simulink model "springmassdamper"  (R2019a)
settings: Solver=ode4  StartTime=0.0  StopTime=5  FixedStep=0.001  RelTol=1e-3
values from neighbouring files (symbols this model uses):
  c = 2 * m * nat_f * 0.05    [smyth_project_2.m]
  k = 19990    [smyth_project_2.m]
  m = 23    [smyth_project_2.m]
  nat_f = sqrt(k/m)    [smyth_project_2.m]
  run_case = 5    [smyth_project_2.m]
  x0 = 0    [smyth_project_2.m]
settings Model: Creator=crsmyth  LastModifiedBy=Ross

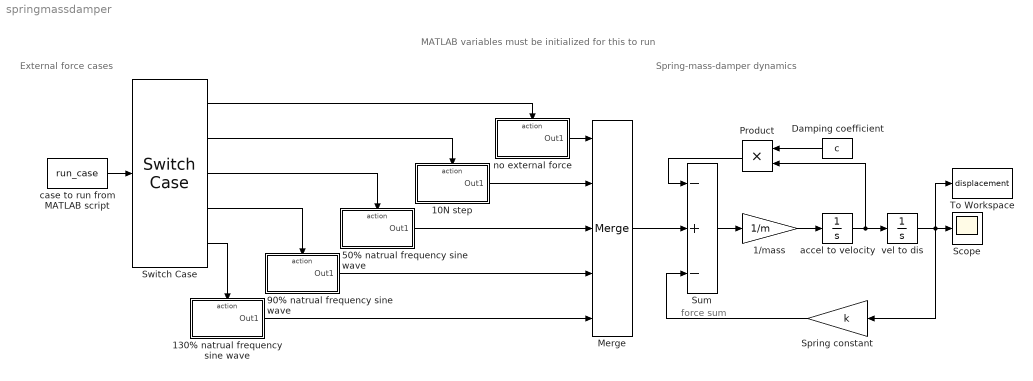
== system springmassdamper ==
  note: MATLAB variables must be initialized for this to run
  note: Spring-mass-damper dynamics
  note: External force cases
  note: force sum
  1/mass : Gain  Gain=1/m
  10N step : Subsystem  TreatAsAtomicUnit=on
  130% natrual frequency sine wave : Subsystem  TreatAsAtomicUnit=on
  50% natrual frequency sine wave : Subsystem  TreatAsAtomicUnit=on
  90% natrual frequency sine wave : Subsystem  TreatAsAtomicUnit=on
  Damping coefficient : Constant  Value=c
  Merge : Merge  Inputs=5
  Product : Product
  Scope : Scope
  Spring constant : Gain  Gain=k
  Sum : Sum  Inputs=-+-
  Switch Case : SwitchCase  CaseConditions={1, 2, 3, 4, 5}  ShowDefaultCase=off
  To Workspace : ToWorkspace  VariableName=displacement  SampleTime=-1
      settings: Save2DSignal=2-D array (concatenate along first dimension)
  accel to velocity : Integrator
  case to run from MATLAB script : Constant  Value=run_case
  no external force : Subsystem  TreatAsAtomicUnit=on
  vel to dis : Integrator  InitialCondition=x0
  wires:
  Sum/1 -> 1/mass/1
  vel to dis/1 -> Scope/1, Spring constant/1, To Workspace/1
  Merge/1 -> Sum/2
  accel to velocity/1 -> Product/2, vel to dis/1
  1/mass/1 -> accel to velocity/1
  Spring constant/1 -> Sum/3
  Switch Case/1 -> no external force/Action
  case to run from MATLAB script/1 -> Switch Case/1
  no external force/1(Out1) -> Merge/1
  10N step/1(Out1) -> Merge/2
  Switch Case/2 -> 10N step/Action
  50% natrual frequency sine wave/1(Out1) -> Merge/3
  Switch Case/3 -> 50% natrual frequency sine wave/Action
  90% natrual frequency sine wave/1(Out1) -> Merge/4
  Switch Case/4 -> 90% natrual frequency sine wave/Action
  130% natrual frequency sine wave/1(Out1) -> Merge/5
  Switch Case/5 -> 130% natrual frequency sine wave/Action
  Product/1 -> Sum/1
  Damping coefficient/1 -> Product/1

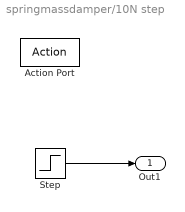
== system springmassdamper/10N step ==
  Action Port : ActionPort  ActionPortLabel=case [ 2 ]:
  Step : Step  Time=0  After=10  SampleTime=0
  Out1 : Outport
  wires:
  Step/1 -> Out1/1

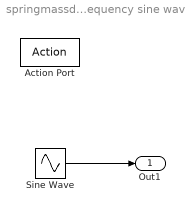
== system springmassdamper/130% natrual frequency sine wave ==
  Action Port : ActionPort  ActionPortLabel=case [ 5 ]:
  Sine Wave : Sin  Amplitude=5  Frequency=nat_f * 1.3  SampleTime=0
  Out1 : Outport
  wires:
  Sine Wave/1 -> Out1/1

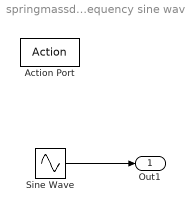
== system springmassdamper/50% natrual frequency sine wave ==
  Action Port : ActionPort  ActionPortLabel=case [ 3 ]:
  Sine Wave : Sin  Amplitude=5  Frequency=nat_f * 0.5  SampleTime=0
  Out1 : Outport
  wires:
  Sine Wave/1 -> Out1/1

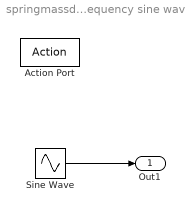
== system springmassdamper/90% natrual frequency sine wave ==
  Action Port : ActionPort  ActionPortLabel=case [ 4 ]:
  Sine Wave : Sin  Amplitude=5  Frequency=nat_f * 0.9  SampleTime=0
  Out1 : Outport
  wires:
  Sine Wave/1 -> Out1/1

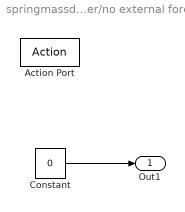
== system springmassdamper/no external force ==
  Action Port : ActionPort  ActionPortLabel=case [ 1 ]:
  Constant : Constant  Value=0
  Out1 : Outport
  wires:
  Constant/1 -> Out1/1
